simulink model "TV_2020_v1_TCELDAS_YAW_1_FUNregenerativa_ETAS"  (R2017b)
settings: Solver=ode3  StartTime=0  StopTime=10  FixedStep=0.05  RelTol=1e-3  EnableMultiTasking=on
(part 1 of 5)
settings Model: Creator=Manuel Montesinos  LastModifiedBy=Eric
settings DataIOCC: LimitDataPoints=on  SaveFormat=Array
settings OptimizationCC: LifeSpan=inf
settings DebuggingCC: SFUnexpectedBacktrackingDiag=warning  SFNoUnconditionalDefaultTransitionDiag=warning  SFExecutionAtInitializationDiag=none
settings HardwareCC: ProdBitPerPointer=32  ProdBitPerSizeT=32  ProdBitPerPtrDiffT=32  ProdLargestAtomicFloat=None  ProdIntDivRoundTo=Undefined  ProdEndianess=Unspecified  ProdWordSize=32  ProdHWDeviceType=32-bit Generic
settings ModelReferenceCC: PropagateSignalLabelsOutOfModel=off
settings CodeAppCC: StateflowObjectComments=on
settings GRTTargetCC: TargetLangStandard=C89/C90 (ANSI)
settings ConfigComp: CovMetricSettings=dw  CovSaveCumulativeToWorkspaceVar=on  CovSaveSingleToWorkspaceVar=on  CovExternalEMLEnable=off

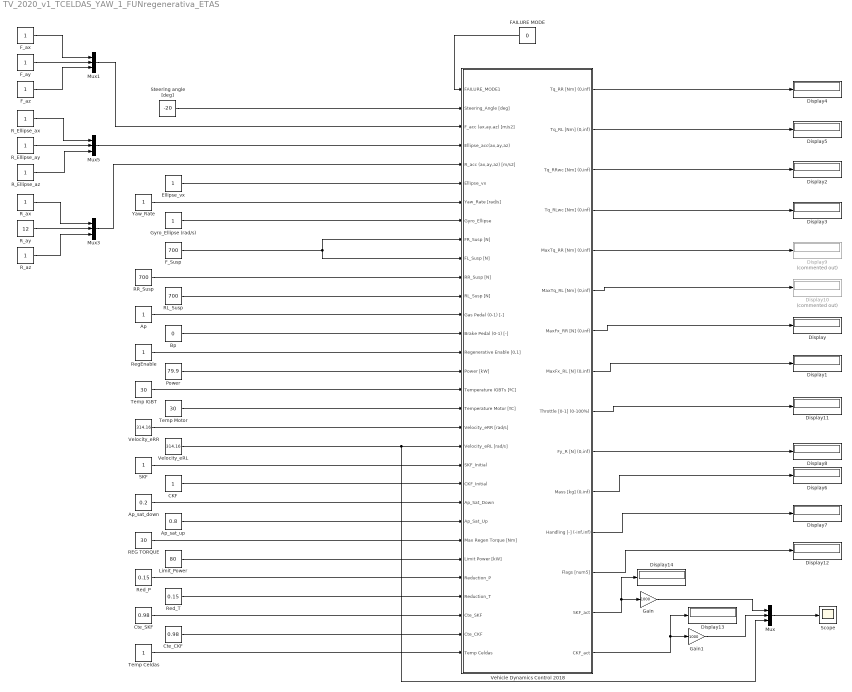
== system TV_2020_v1_TCELDAS_YAW_1_FUNregenerativa_ETAS ==
  Ap : Constant
  Ap_sat_down : Constant  Value=0.2
  Ap_sat_up : Constant  Value=0.8
  Bp : Constant  Value=0
  CKF : Constant
  Cte_CKF : Constant  Value=0.98
  Cte_SKF : Constant  Value=0.98
  Display{,1..8,11..14} (13 alike) : Display
  Display10 : Display  Commented=on
  Display9 : Display  Commented=on
  Ellipse_vx : Constant
  FAILURE MODE : Constant  Value=0
  F_Susp : Constant  Value=700
  F_ax : Constant
  F_ay : Constant
  F_az : Constant
  Gain : Gain  Gain=1000
  Gain1 : Gain  Gain=1000
  Gyro_Ellipse (rad/s) : Constant
  Limit_Power : Constant  Value=80
  Mux{,1,3,5} (4 alike) : Mux  Inputs=3
  Power : Constant  Value=79.9
  REG TORQUE : Constant  Value=30
  RL_Susp : Constant  Value=700
  RR_Susp : Constant  Value=700
  R_Ellipse_ax : Constant
  R_Ellipse_ay : Constant
  R_Ellipse_az : Constant
  R_ax : Constant
  R_ay : Constant  Value=12
  R_az : Constant
  Red_P : Constant  Value=0.15
  Red_T : Constant  Value=0.15
  RegEnable : Constant
  SKF : Constant
  Scope : Scope
  Steering angle [deg] : Constant  Value=-20
  Temp Celdas : Constant
  Temp IGBT : Constant  Value=30
  Temp Motor : Constant  Value=30
  Vehicle Dynamics Control 2018 : Subsystem
  Velocity_eRL : Constant  Value=314.16
  Velocity_eRR : Constant  Value=314.16
  Yaw_Rate : Constant
  wires:
  FAILURE MODE/1 -> Vehicle Dynamics Control 2018/1(FAILURE_MODE1)
  Vehicle Dynamics Control 2018/1(Tq_RR [Nm] (0,inf)) -> Display4/1
  Vehicle Dynamics Control 2018/2(Tq_RL [Nm] (0,inf)) -> Display5/1
  Mux3/1 -> Vehicle Dynamics Control 2018/5(R_acc (ax,ay,az) [m/s2])
  RegEnable/1 -> Vehicle Dynamics Control 2018/15(Regenerative Enable [0,1])
  Velocity_eRL/1 -> Vehicle Dynamics Control 2018/20(Velocity_eRL [rad/s]), Mux/3
  SKF/1 -> Vehicle Dynamics Control 2018/21(SKF_Initial)
  CKF/1 -> Vehicle Dynamics Control 2018/22(CKF_Initial)
  REG TORQUE/1 -> Vehicle Dynamics Control 2018/25(Max Regen Torque [Nm])
  Limit_Power/1 -> Vehicle Dynamics Control 2018/26(Limit Power [kW])
  Red_T/1 -> Vehicle Dynamics Control 2018/28(Reduction_T)
  Red_P/1 -> Vehicle Dynamics Control 2018/27(Reduction_P)
  F_Susp/1 -> Vehicle Dynamics Control 2018/9(FR_Susp [N]), Vehicle Dynamics Control 2018/10(FL_Susp [N])
  Vehicle Dynamics Control 2018/7(MaxFx_RR [N] (0,inf)) -> Display/1
  Vehicle Dynamics Control 2018/8(MaxFx_RL [N] (0,inf)) -> Display1/1
  Vehicle Dynamics Control 2018/3(Tq_RRwc [Nm] (0,inf)) -> Display2/1
  Vehicle Dynamics Control 2018/4(Tq_RLwc [Nm] (0,inf)) -> Display3/1
  Vehicle Dynamics Control 2018/6(MaxTq_RL [Nm] (0,inf)) -> Display10/1
  Vehicle Dynamics Control 2018/5(MaxTq_RR [Nm] (0,inf)) -> Display9/1
  Vehicle Dynamics Control 2018/10(Fy_R [N] (0,inf)) -> Display8/1
  Steering angle [deg]/1 -> Vehicle Dynamics Control 2018/2(Steering_Angle [deg])
  RR_Susp/1 -> Vehicle Dynamics Control 2018/11(RR_Susp [N])
  RL_Susp/1 -> Vehicle Dynamics Control 2018/12(RL_Susp [N])
  Bp/1 -> Vehicle Dynamics Control 2018/14(Brake Pedal (0-1) [-])
  Ap/1 -> Vehicle Dynamics Control 2018/13(Gas Pedal (0-1) [-])
  Ap_sat_down/1 -> Vehicle Dynamics Control 2018/23(Ap_Sat_Down)
  Vehicle Dynamics Control 2018/11(Mass [kg] (0,inf)) -> Display6/1
  Vehicle Dynamics Control 2018/12(Handling [-] (-inf,inf)) -> Display7/1
  Mux1/1 -> Vehicle Dynamics Control 2018/3(F_acc (ax,ay,az) [m/s2])
  Temp IGBT/1 -> Vehicle Dynamics Control 2018/17(Temperature IGBTs [ºC])
  Power/1 -> Vehicle Dynamics Control 2018/16(Power [kW])
  Temp Motor/1 -> Vehicle Dynamics Control 2018/18(Temperature Motor [ºC])
  Ap_sat_up/1 -> Vehicle Dynamics Control 2018/24(Ap_Sat_Up)
  Vehicle Dynamics Control 2018/9(Throttle [0-1] (0-100%)) -> Display11/1
  Vehicle Dynamics Control 2018/13(Flags [num5]) -> Display12/1
  Cte_SKF/1 -> Vehicle Dynamics Control 2018/29(Cte_SKF)
  Cte_CKF/1 -> Vehicle Dynamics Control 2018/30(Cte_CKF)
  Vehicle Dynamics Control 2018/15(CKF_act) -> Display13/1, Gain1/1
  Vehicle Dynamics Control 2018/14(SKF_act) -> Display14/1, Gain/1
  Mux/1 -> Scope/1
  Gain/1 -> Mux/1
  Gain1/1 -> Mux/2
  Yaw_Rate/1 -> Vehicle Dynamics Control 2018/7(Yaw_Rate [rad/s])
  F_ax/1 -> Mux1/1
  F_ay/1 -> Mux1/2
  F_az/1 -> Mux1/3
  R_ax/1 -> Mux3/1
  R_ay/1 -> Mux3/2
  R_az/1 -> Mux3/3
  Velocity_eRR/1 -> Vehicle Dynamics Control 2018/19(Velocity_eRR [rad/s])
  Mux5/1 -> Vehicle Dynamics Control 2018/4(Ellipse_acc(ax,ay,az))
  R_Ellipse_ay/1 -> Mux5/2
  R_Ellipse_ax/1 -> Mux5/1
  R_Ellipse_az/1 -> Mux5/3
  Ellipse_vx/1 -> Vehicle Dynamics Control 2018/6(Ellipse_vx)
  Gyro_Ellipse (rad/s)/1 -> Vehicle Dynamics Control 2018/8(Gyro_Ellipse)
  Temp Celdas/1 -> Vehicle Dynamics Control 2018/31(Temp Celdas)

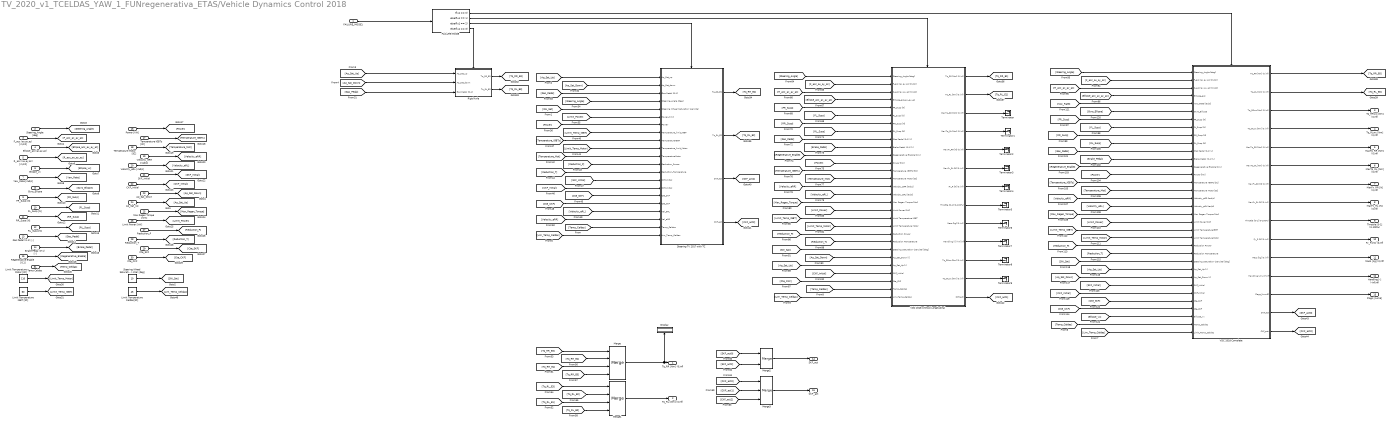
== system TV_2020_v1_TCELDAS_YAW_1_FUNregenerativa_ETAS/Vehicle Dynamics Control 2018 ==
  FAILURE_MODE1 : Inport
  Steering_Angle [deg] : Inport  Port=2
  F_acc (ax,ay,az) [m/s2] : Inport  Port=3
  Ellipse_acc(ax,ay,az) : Inport  Port=4
  R_acc (ax,ay,az) [m/s2] : Inport  Port=5
  Ellipse_vx : Inport  Port=6
  Yaw_Rate [rad/s] : Inport  Port=7
  Gyro_Ellipse : Inport  Port=8
  FR_Susp [N] : Inport  Port=9
  FL_Susp [N] : Inport  Port=10
  RR_Susp [N] : Inport  Port=11
  RL_Susp [N] : Inport  Port=12
  Gas Pedal (0-1) [-] : Inport  Port=13
  Brake Pedal (0-1) [-] : Inport  Port=14
  Regenerative Enable [0,1] : Inport  Port=15
  Power [kW] : Inport  Port=16
  Temperature IGBTs [ºC] : Inport  Port=17
  Temperature Motor [ºC] : Inport  Port=18
  Velocity_eRR [rad/s] : Inport  Port=19
  Velocity_eRL [rad/s] : Inport  Port=20
  SKF_Initial : Inport  Port=21
  CKF_Initial : Inport  Port=22
  Ap_Sat_Down : Inport  Port=23
  Ap_Sat_Up : Inport  Port=24
  Max Regen Torque [Nm] : Inport  Port=25
  Limit Power [kW] : Inport  Port=26
  Reduction_P : Inport  Port=27
  Reduction_T : Inport  Port=28
  Cte_SKF : Inport  Port=29
  Cte_CKF : Inport  Port=30
  Temp Celdas : Inport  Port=31
  Display : Display
  FAILURE MODE : If  IfExpression=u1 == 0  ElseIfExpressions=u1 == 1, u1 == 2, u1 == 3  ShowElse=off
  Limit Temperature Celdas[ºC] : Constant  Value=45
  Limit Temperature IGBT [ºC] : Constant  Value=60
  Limit Temperature Motor [ºC] : Constant  Value=110
  Merge : Merge  Inputs=4
  Merge1 : Merge  Inputs=4
  Merge2 : Merge
  Merge3 : Merge  Inputs=3
  Rigid Axle : Subsystem  TreatAsAtomicUnit=on
  Steering TV 2017 with TC : Subsystem  TreatAsAtomicUnit=on
  "Steering Wheel Saturation (per site) [deg] " : Constant  Value=10
  Terminator{,1..9} (10 alike) : Terminator
  VDC 2018 Complete : Subsystem  TreatAsAtomicUnit=on
  VDC 2018 without Longitudinal : Subsystem  TreatAsAtomicUnit=on
  Tq_RR [Nm] (0,inf) : Outport
  Tq_RL [Nm] (0,inf) : Outport  Port=2
  Tq_RRwc [Nm] (0,inf) : Outport  Port=3
  Tq_RLwc [Nm] (0,inf) : Outport  Port=4
  MaxTq_RR [Nm] (0,inf) : Outport  Port=5
  MaxTq_RL [Nm] (0,inf) : Outport  Port=6
  MaxFx_RR [N] (0,inf) : Outport  Port=7
  MaxFx_RL [N] (0,inf) : Outport  Port=8
  Throttle [0-1] (0-100%) : Outport  Port=9
  Fy_R [N] (0,inf) : Outport  Port=10
  Mass [kg] (0,inf) : Outport  Port=11
  Handling [-] (-inf,inf) : Outport  Port=12
  Flags [num5] : Outport  Port=13
  SKF_act : Outport  Port=14
  CKF_act : Outport  Port=15
  wires:
  Merge1/1 -> Tq_RL [Nm] (0,inf)/1
  Merge/1 -> Display/1, Tq_RR [Nm] (0,inf)/1
  Ap_Sat_Down/1 -> [Ap_Sat_Down]
  "Steering Wheel Saturation (per site) [deg] "/1 -> [SW_Sat]
  [Ap_Sat_Up] -> Rigid Axle/1("Ap_Sat_up ")
  [Ap_Sat_Down] -> Rigid Axle/2(Ap_Sat_down)
  VDC 2018 Complete/4(Tq_RLwc [Nm] (0,inf)) -> Tq_RLwc [Nm] (0,inf)/1
  VDC 2018 Complete/3(Tq_RRwc [Nm] (0,inf)) -> Tq_RRwc [Nm] (0,inf)/1
  VDC 2018 Complete/5(MaxTq_RR [Nm] (0,inf)) -> MaxTq_RR [Nm] (0,inf)/1
  VDC 2018 Complete/6(MaxTq_RL [Nm] (0,inf)) -> MaxTq_RL [Nm] (0,inf)/1
  VDC 2018 Complete/7(MaxFx_RR [N] (0,inf)) -> MaxFx_RR [N] (0,inf)/1
  VDC 2018 Complete/8(MaxFx_RL [N] (0,inf)) -> MaxFx_RL [N] (0,inf)/1
  VDC 2018 Complete/9(Throttle [0-1] (0-100%)) -> Throttle [0-1] (0-100%)/1
  VDC 2018 Complete/10(Fy_R [N] (0,inf)) -> Fy_R [N] (0,inf)/1
  VDC 2018 Complete/11(Mass [kg] (0,inf)) -> Mass [kg] (0,inf)/1
  VDC 2018 Complete/12(Handling [-] (-inf,inf)) -> Handling [-] (-inf,inf)/1
  VDC 2018 without Longitudinal/3(MaxTq_RR [Nm] (0,inf)) -> Terminator/1
  VDC 2018 without Longitudinal/4(MaxTq_RL [Nm] (0,inf)) -> Terminator1/1
  VDC 2018 without Longitudinal/5(MaxFx_RR [N] (0,inf)) -> Terminator2/1
  VDC 2018 without Longitudinal/6(MaxFx_RL [N] (0,inf)) -> Terminator3/1
  VDC 2018 without Longitudinal/7(Fy_R [N] (0,inf)) -> Terminator4/1
  VDC 2018 without Longitudinal/8(Throttle [0-1] (0-100%)) -> Terminator5/1
  VDC 2018 without Longitudinal/9(Mass [kg] (0,inf)) -> Terminator6/1
  VDC 2018 without Longitudinal/10(Handling [-] (-inf,inf)) -> Terminator7/1
  VDC 2018 without Longitudinal/11(Tq_RRwc [Nm] (0,inf)) -> Terminator8/1
  VDC 2018 without Longitudinal/12(Tq_RLwc [Nm] (0,inf)) -> Terminator9/1
  Ap_Sat_Up/1 -> [Ap_Sat_Up]
  VDC 2018 Complete/13(Flags_[num5]) -> Flags [num5]/1
  Merge2/1 -> SKF_act/1
  Merge3/1 -> CKF_act/1
  Steering_Angle [deg]/1 -> [Steering_Angle]
  F_acc (ax,ay,az) [m/s2]/1 -> [F_acc_ax_ay_az]
  Ellipse_acc(ax,ay,az)/1 -> [Ellipse_acc_ax_ay_az]
  R_acc (ax,ay,az) [m/s2]/1 -> [R_acc_ax_ay_az]
  Ellipse_vx/1 -> [Ellipse_vx]
  Yaw_Rate [rad/s]/1 -> [Yaw_Rate]
  Gyro_Ellipse/1 -> [Gyro_Ellipse]
  FR_Susp [N]/1 -> [FR_Susp]
  FL_Susp [N]/1 -> [FL_Susp]
  RR_Susp [N]/1 -> [RR_Susp]
  RL_Susp [N]/1 -> [RL_Susp]
  Gas Pedal (0-1) [-]/1 -> [Gas_Pedal]
  Brake Pedal (0-1) [-]/1 -> [Brake_Pedal]
  Regenerative Enable [0,1]/1 -> [Regenerative_Enable]
  Power [kW]/1 -> [Power]
  Temperature IGBTs [ºC]/1 -> [Temperature_IGBTs]
  Temperature Motor [ºC]/1 -> [Temperature_Mot]
  Velocity_eRR [rad/s]/1 -> [Velocity_eRR]
  Velocity_eRL [rad/s]/1 -> [Velocity_eRL]
  SKF_Initial/1 -> [SKF_Initial]
  CKF_Initial/1 -> [CKF_Initial]
  Max Regen Torque [Nm]/1 -> [Max_Regen_Torque]
  Limit Power [kW]/1 -> [Limit_Power]
  Reduction_P/1 -> [Reduction_P]
  Reduction_T/1 -> [Reduction_T]
  Cte_SKF/1 -> [Cte_SKF]
  Cte_CKF/1 -> [Cte_CKF]
  [Gas_Pedal] -> Rigid Axle/3(Gas Pedal [0-1])
  [Ap_Sat_Up] -> Steering TV 2017 with TC/1("Ap_Sat_up ")
  [Ap_Sat_Down] -> Steering TV 2017 with TC/2(Ap_Sat_down)
  [Gas_Pedal] -> Steering TV 2017 with TC/3(Gas Pedal [0-1])
  [Steering_Angle] -> Steering TV 2017 with TC/4(Steering_Angle [deg])
  [SW_Sat] -> Steering TV 2017 with TC/5("Steering Wheel Saturation (per site) ")
  [Limit_Power] -> Steering TV 2017 with TC/6(Power_limit)
  [Power] -> Steering TV 2017 with TC/7(Power)
  Limit Temperature Motor [ºC]/1 -> [Limit_Temp_Motor]
  Limit Temperature IGBT [ºC]/1 -> [Limit_Temp_IGBT]
  [Limit_Temp_Motor] -> Steering TV 2017 with TC/10(Temperature_limit_Motor)
  [Limit_Temp_IGBT] -> Steering TV 2017 with TC/8(Temperature_limit_IGBT)
  [Temperature_IGBTs] -> Steering TV 2017 with TC/9(TemperatureIGBT)
  [Temperature_Mot] -> Steering TV 2017 with TC/11(TemperatureMotor)
  [Reduction_P] -> Steering TV 2017 with TC/12(Reduction_Power)
  [Reduction_T] -> Steering TV 2017 with TC/13(Reduction_Temperature)
  [SKF_Initial] -> Steering TV 2017 with TC/14(SKF_Initial)
  [CKF_Initial] -> Steering TV 2017 with TC/15(CKF_Initial)
  [Cte_SKF] -> Steering TV 2017 with TC/16(Cte_SKF)
  [Cte_CKF] -> Steering TV 2017 with TC/17(Cte_CKF)
  [Velocity_eRL] -> Steering TV 2017 with TC/18(Vel_eRL)
  [Velocity_eRR] -> Steering TV 2017 with TC/19(Vel_eRR)
  Rigid Axle/1(Tq_RR_E3) -> [Tq_RR_E3]
  Rigid Axle/2(Tq_RL_E3) -> [Tq_RL_E3]
  [Tq_RL_E3] -> Merge1/1
  [Tq_RR_E3] -> Merge/1
  Steering TV 2017 with TC/1(Tq_RR_E2) -> [Tq_RR_E2]
  Steering TV 2017 with TC/2(Tq_RL_E2) -> [Tq_RL_E2]
  [Tq_RL_E2] -> Merge1/2
  [Tq_RR_E2] -> Merge/2
  VDC 2018 without Longitudinal/2(Tq_RL [Nm] (0,inf)) -> [Tq_RL_E1]
  VDC 2018 without Longitudinal/1(Tq_RR [Nm] (0,inf)) -> [Tq_RR_E1]
  [Tq_RR_E1] -> Merge/3
  [Tq_RL_E1] -> Merge1/3
  VDC 2018 Complete/1(Tq_RR [Nm] (0,inf)) -> [Tq_RR_E0]
  VDC 2018 Complete/2(Tq_RL [Nm] (0,inf)) -> [Tq_RL_E0]
  [Tq_RR_E0] -> Merge/4
  [Tq_RL_E0] -> Merge1/4
  Steering TV 2017 with TC/3(SKF_act) -> [SKF_act2]
  Steering TV 2017 with TC/4(CKF_act) -> [CKF_act2]
  VDC 2018 without Longitudinal/13(CKF_act) -> [CKF_act1]
  VDC 2018 Complete/14(SKF_act) -> [SKF_act0]
  VDC 2018 Complete/15(CKF_act) -> [CKF_act0]
  [CKF_act1] -> Merge3/2
  [CKF_act0] -> Merge3/1
  [CKF_act2] -> Merge3/3
  [SKF_act0] -> Merge2/1
  [SKF_act2] -> Merge2/2
  [Steering_Angle] -> VDC 2018 without Longitudinal/1(Steering_Angle [deg])
  [F_acc_ax_ay_az] -> VDC 2018 without Longitudinal/2(F_acc (ax,ay,az) [m/s2])
  [Ellipse_acc_ax_ay_az] -> VDC 2018 without Longitudinal/4(Ellipse_acc_ax_ay_az)
  [R_acc_ax_ay_az] -> VDC 2018 without Longitudinal/3(R_acc (ax,ay,az) [m/s2])
  [FR_Susp] -> VDC 2018 without Longitudinal/5(FR_Susp [N])
  [FL_Susp] -> VDC 2018 without Longitudinal/6(FL_Susp [N])
  [RR_Susp] -> VDC 2018 without Longitudinal/7(RR_Susp [N])
  [RL_Susp] -> VDC 2018 without Longitudinal/8(RL_Susp [N])
  [Gas_Pedal] -> VDC 2018 without Longitudinal/9(Gas Pedal (0-1) [-])
  [Brake_Pedal] -> VDC 2018 without Longitudinal/10(Brake Pedal (0-1) [-])
  [Regenerative_Enable] -> VDC 2018 without Longitudinal/11(Regenerative Enable [0,1])
  [Power] -> VDC 2018 without Longitudinal/12(Power [kW])
  [Temperature_IGBTs] -> VDC 2018 without Longitudinal/13(Temperature IGBTs [ºC])
  [Temperature_Mot] -> VDC 2018 without Longitudinal/14(Temperature Motor [ºC])
  [Velocity_eRR] -> VDC 2018 without Longitudinal/15(Velocity_eRR [rad/s])
  [Velocity_eRL] -> VDC 2018 without Longitudinal/16(Velocity_eRL [rad/s])
  [Max_Regen_Torque] -> VDC 2018 without Longitudinal/17(Max Regen Torque [Nm])
  [Limit_Power] -> VDC 2018 without Longitudinal/18(Limit Power [kW])
  [Limit_Temp_IGBT] -> VDC 2018 without Longitudinal/19(Limit Temperature IGBT)
  [Limit_Temp_Motor] -> VDC 2018 without Longitudinal/20(Limit Temperature Motor)
  [Cte_CKF] -> VDC 2018 without Longitudinal/27(Cte_CKF)
  [Reduction_P] -> VDC 2018 without Longitudinal/21(Reduction Power)
  [Reduction_T] -> VDC 2018 without Longitudinal/22(Reduction Temperature)
  [Ap_Sat_Up] -> VDC 2018 without Longitudinal/25(Ap_Sat_Up [-])
  [Ap_Sat_Down] -> VDC 2018 without Longitudinal/24(Ap_Sat_Down [-])
  [SW_Sat] -> VDC 2018 without Longitudinal/23(Steering Saturation (per site) [deg])
  [CKF_Initial] -> VDC 2018 without Longitudinal/26(CKF_Initial)
  [Steering_Angle] -> VDC 2018 Complete/1(Steering_Angle [deg])
  [F_acc_ax_ay_az] -> VDC 2018 Complete/2(F_acc (ax,ay,az) [m/s2])
  [R_acc_ax_ay_az] -> VDC 2018 Complete/3(R_acc (ax,ay,az) [m/s2])
  [Ellipse_acc_ax_ay_az] -> VDC 2018 Complete/4(Ellipse_acc)
  [FR_Susp] -> VDC 2018 Complete/7(FR_Susp [N])
  [FL_Susp] -> VDC 2018 Complete/8(FL_Susp [N])
  [RR_Susp] -> VDC 2018 Complete/9(RR_Susp [N])
  [RL_Susp] -> VDC 2018 Complete/10(RL_Susp [N])
  [Gas_Pedal] -> VDC 2018 Complete/11(Gas Pedal (0-1) [-])
  [Brake_Pedal] -> VDC 2018 Complete/12(Brake Pedal (0-1) [-])
  [Power] -> VDC 2018 Complete/14(Power [kW])
  [Regenerative_Enable] -> VDC 2018 Complete/13(Regenerative Enable [0,1])
  [Temperature_IGBTs] -> VDC 2018 Complete/15(Temperature IGBTs [ºC])
  [Temperature_Mot] -> VDC 2018 Complete/16(Temperature Motor [ºC])
  [Velocity_eRR] -> VDC 2018 Complete/17(Velocity_eRR [rad/s])
  [Velocity_eRL] -> VDC 2018 Complete/18(Velocity_eRL [rad/s])
  [Max_Regen_Torque] -> VDC 2018 Complete/19(Max Regen Torque [Nm])
  [Limit_Power] -> VDC 2018 Complete/20(Limit Power [kW])
  [Limit_Temp_IGBT] -> VDC 2018 Complete/21(Limit TemperatureIGBT)
  [Limit_Temp_Motor] -> VDC 2018 Complete/22(Limit TemperatureMotor)
  [Reduction_P] -> VDC 2018 Complete/23(Reduction Power)
  [Reduction_T] -> VDC 2018 Complete/24(Reduction Temperature)
  [SW_Sat] -> VDC 2018 Complete/25(Steering Saturation (per site) [deg])
  [Ap_Sat_Down] -> VDC 2018 Complete/27(Ap_Sat_Down [-])
  [Ap_Sat_Up] -> VDC 2018 Complete/26(Ap_Sat_Up [-])
  [CKF_Initial] -> VDC 2018 Complete/29(CKF_Initial)
  [Yaw_Rate] -> VDC 2018 Complete/5(Yaw_Rate [rad/s])
  [Gyro_Ellipse] -> VDC 2018 Complete/6(Gyro_Ellipse)
  [Cte_CKF] -> VDC 2018 Complete/31(Cte_CKF)
  [Cte_SKF] -> VDC 2018 Complete/30(Cte_SKF)
  [SKF_Initial] -> VDC 2018 Complete/28(SKF_Initial)
  [Ellipse_vx] -> VDC 2018 Complete/32(Ellipse_vx)
  FAILURE MODE/1 -> VDC 2018 Complete/Action
  FAILURE_MODE1/1 -> FAILURE MODE/1
  FAILURE MODE/2 -> VDC 2018 without Longitudinal/Action
  FAILURE MODE/3 -> Steering TV 2017 with TC/Action
  FAILURE MODE/4 -> Rigid Axle/Action
  Temp Celdas/1 -> [Temp_Celdas]
  Limit Temperature Celdas[ºC]/1 -> [Lim_Temp_Celdas]
  [Temp_Celdas] -> Steering TV 2017 with TC/20(Temp_Celdas)
  [Lim_Temp_Celdas] -> Steering TV 2017 with TC/21(Lim_Temp_Celdas)
  [Temp_Celdas] -> VDC 2018 without Longitudinal/28(Temp_Celdas)
  [Lim_Temp_Celdas] -> VDC 2018 without Longitudinal/29(Lim_Temp_Celdas)
  [Temp_Celdas] -> VDC 2018 Complete/33(Temp_Celdas)
  [Lim_Temp_Celdas] -> VDC 2018 Complete/34(Limit_Temp_Celdas)

== system TV_2020_v1_TCELDAS_YAW_1_FUNregenerativa_ETAS/Vehicle Dynamics Control 2018/Rigid Axle ==
  "Ap_Sat_up " : Inport
  Ap_Sat_down : Inport  Port=2
  Gas Pedal [0-1] : Inport  Port=3
  Action Port : ActionPort
  Accelerating : Subsystem
  Torque_RL [Nm] : Constant  Value=60
  Torque_RR [Nm] : Constant  Value=60
  Tq_RR_E3 : Outport
  Tq_RL_E3 : Outport  Port=2
  wires:
  Torque_RR [Nm]/1 -> Accelerating/4(Tq_RR)
  Torque_RL [Nm]/1 -> Accelerating/5("Tq_RL ")
  Accelerating/2(Tq_RL) -> Tq_RL_E3/1
  Accelerating/1("Tq_RR ") -> Tq_RR_E3/1
  Gas Pedal [0-1]/1 -> Accelerating/1(Ap)
  "Ap_Sat_up "/1 -> Accelerating/2("Ap_Sat_up ")
  Ap_Sat_down/1 -> Accelerating/3(Ap_Sat_down)

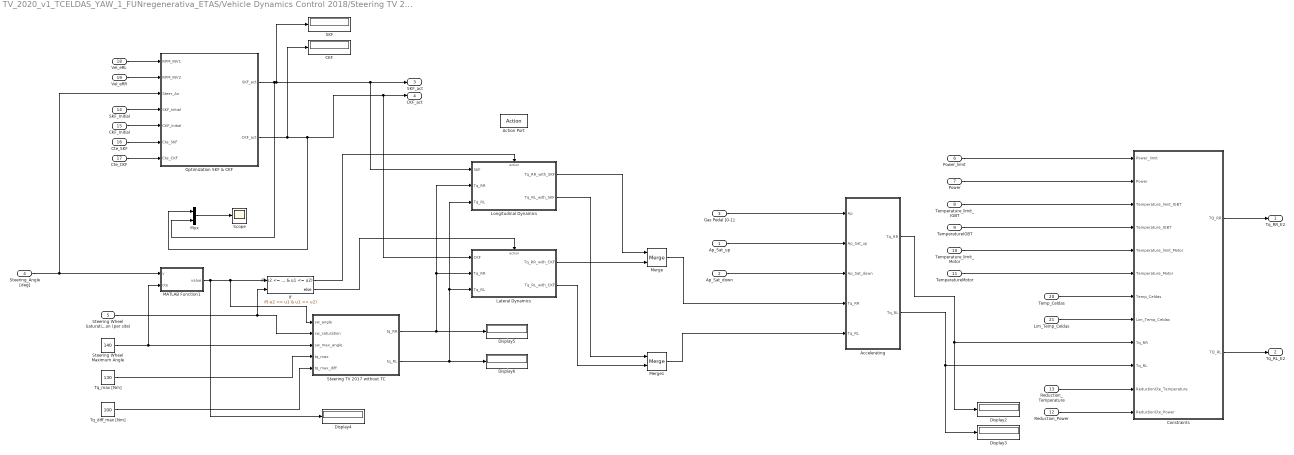
== system TV_2020_v1_TCELDAS_YAW_1_FUNregenerativa_ETAS/Vehicle Dynamics Control 2018/Steering TV 2017 with TC ==
  "Ap_Sat_up " : Inport
  Ap_Sat_down : Inport  Port=2
  Gas Pedal [0-1] : Inport  Port=3
  Steering_Angle [deg] : Inport  Port=4
  "Steering Wheel Saturation (per site) " : Inport  Port=5
  Power_limit : Inport  Port=6
  Power : Inport  Port=7
  Temperature_limit_IGBT : Inport  Port=8
  TemperatureIGBT : Inport  Port=9
  Temperature_limit_Motor : Inport  Port=10
  TemperatureMotor : Inport  Port=11
  Reduction_Power : Inport  Port=12
  Reduction_Temperature : Inport  Port=13
  SKF_Initial : Inport  Port=14
  CKF_Initial : Inport  Port=15
  Cte_SKF : Inport  Port=16
  Cte_CKF : Inport  Port=17
  Vel_eRL : Inport  Port=18
  Vel_eRR : Inport  Port=19
  Temp_Celdas : Inport  Port=20
  Lim_Temp_Celdas : Inport  Port=21
  Action Port : ActionPort
  Accelerating : Subsystem
  CKF : Display
  Constraints : Subsystem
  Display{2..6} (5 alike) : Display
  If : If  NumInputs=2  IfExpression=-u2 <= u1 & u1 <= u2
  Lateral Dynamics : Subsystem  TreatAsAtomicUnit=on
  Longitudinal Dynamics : Subsystem  TreatAsAtomicUnit=on
  MATLAB Function1 : MATLAB Function  TreatAsAtomicUnit=on
  Merge : Merge
  Merge1 : Merge
  Mux : Mux  Inputs=2
  Optimization SKF & CKF : Subsystem
  SKF : Display
  Scope : Scope
  Steering TV 2017 without TC : MATLAB Function  TreatAsAtomicUnit=on
  Steering Wheel Maximum Angle : Constant  Value=140
  Tq_diff_max [Nm] : Constant  Value=100
  Tq_max [Nm] : Constant  Value=130
  Tq_RR_E2 : Outport
  Tq_RL_E2 : Outport  Port=2
  SKF_act : Outport  Port=3
  CKF_act : Outport  Port=4
  wires:
  Gas Pedal [0-1]/1 -> Accelerating/1(Ap)
  "Ap_Sat_up "/1 -> Accelerating/2("Ap_Sat_up ")
  Ap_Sat_down/1 -> Accelerating/3(Ap_Sat_down)
  Tq_max [Nm]/1 -> Steering TV 2017 without TC/4(tq_max)
  Tq_diff_max [Nm]/1 -> Steering TV 2017 without TC/5(tq_max_diff)
  Steering Wheel Maximum Angle/1 -> Steering TV 2017 without TC/3(sw_max_angle), MATLAB Function1/2(cte)
  "Steering Wheel Saturation (per site) "/1 -> If/2, Steering TV 2017 without TC/2(sw_saturation)
  Steering TV 2017 without TC/1(tq_RR) -> Display5/1, Longitudinal Dynamics/2(Tq_RR), Lateral Dynamics/2(Tq_RR)
  Steering TV 2017 without TC/2(tq_RL) -> Longitudinal Dynamics/3(Tq_RL), Lateral Dynamics/3(Tq_RL), Display6/1
  Power_limit/1 -> Constraints/1(Power_limit)
  Power/1 -> Constraints/2(Power)
  Temperature_limit_IGBT/1 -> Constraints/3(Temperature_limit_IGBT)
  TemperatureIGBT/1 -> Constraints/4(Temperature_IGBT)
  Reduction_Temperature/1 -> Constraints/11(ReductionCte_Temperature)
  Reduction_Power/1 -> Constraints/12(ReductionCte_Power)
  Constraints/1(TQ_RR) -> Tq_RR_E2/1
  Constraints/2(TQ_RL) -> Tq_RL_E2/1
  Accelerating/2(Tq_RL) -> Display3/1, Constraints/10(Tq_RL)
  Accelerating/1("Tq_RR ") -> Display2/1, Constraints/9(Tq_RR)
  MATLAB Function1/1(value) -> Display4/1, Steering TV 2017 without TC/1(sw_angle), If/1
  Temperature_limit_Motor/1 -> Constraints/5(Temperature_limit_Motor)
  TemperatureMotor/1 -> Constraints/6(Temperature_Motor)
  Optimization SKF & CKF/2(CKF_act) -> CKF/1, Mux/1, Lateral Dynamics/1(CKF), CKF_act/1
  SKF_Initial/1 -> Optimization SKF & CKF/4(SKF_Initial)
  Mux/1 -> Scope/1
  Cte_SKF/1 -> Optimization SKF & CKF/6(Cte_SKF)
  Vel_eRL/1 -> Optimization SKF & CKF/1(RPM_INV1)
  Vel_eRR/1 -> Optimization SKF & CKF/2(RPM_INV2)
  Optimization SKF & CKF/1(SKF_act) -> SKF_act/1, Longitudinal Dynamics/1(SKF), SKF/1, Mux/2
  Steering_Angle [deg]/1 -> MATLAB Function1/1(v), Optimization SKF & CKF/3(Steer_An)
  CKF_Initial/1 -> Optimization SKF & CKF/5(CKF_Initial)
  Cte_CKF/1 -> Optimization SKF & CKF/7(Cte_CKF)
  If/1 -> Longitudinal Dynamics/Action
  Lateral Dynamics/2(Tq_RL_with_CKF) -> Merge1/2
  If/2 -> Lateral Dynamics/Action
  Longitudinal Dynamics/2(Tq_RL_with_SKF) -> Merge1/1
  Longitudinal Dynamics/1(Tq_RR_with_SKF) -> Merge/1
  Lateral Dynamics/1(Tq_RR_with_CKF) -> Merge/2
  Merge/1 -> Accelerating/4(Tq_RR)
  Merge1/1 -> Accelerating/5("Tq_RL ")
  Temp_Celdas/1 -> Constraints/7(Temp_Celdas)
  Lim_Temp_Celdas/1 -> Constraints/8(Lim_Temp_Celdas)

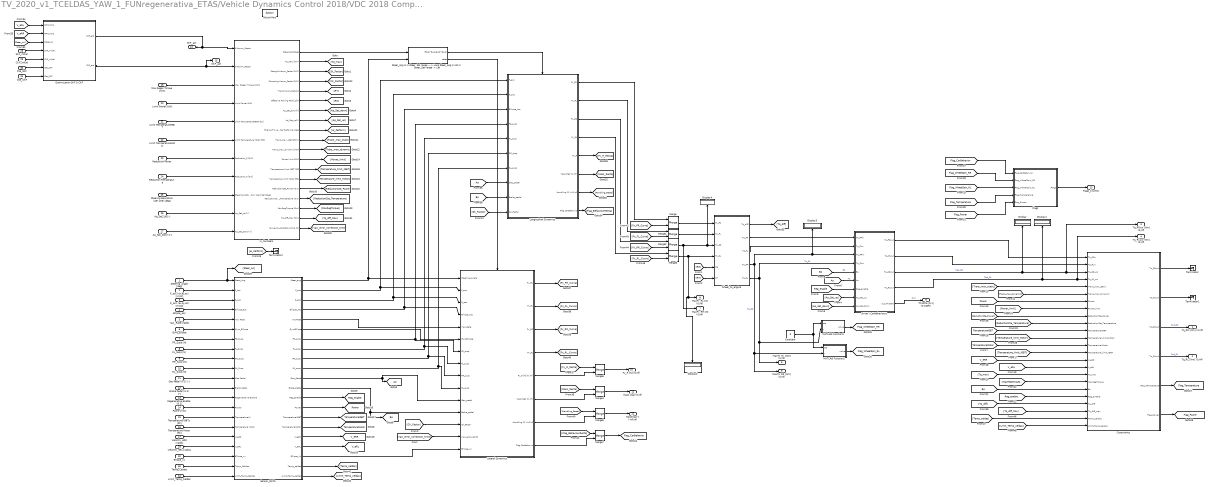
== system TV_2020_v1_TCELDAS_YAW_1_FUNregenerativa_ETAS/Vehicle Dynamics Control 2018/VDC 2018 Complete ==
  Steering_Angle [deg] : Inport
  F_acc (ax,ay,az) [m/s2] : Inport  Port=2
  R_acc (ax,ay,az) [m/s2] : Inport  Port=3
  Ellipse_acc : Inport  Port=4
  Yaw_Rate [rad/s] : Inport  Port=5
  Gyro_Ellipse : Inport  Port=6
  FR_Susp [N] : Inport  Port=7
  FL_Susp [N] : Inport  Port=8
  RR_Susp [N] : Inport  Port=9
  RL_Susp [N] : Inport  Port=10
  Gas Pedal (0-1) [-] : Inport  Port=11
  Brake Pedal (0-1) [-] : Inport  Port=12
  Regenerative Enable [0,1] : Inport  Port=13
  Power [kW] : Inport  Port=14
  Temperature IGBTs [ºC] : Inport  Port=15
  Temperature Motor [ºC] : Inport  Port=16
  Velocity_eRR [rad/s] : Inport  Port=17
  Velocity_eRL [rad/s] : Inport  Port=18
  Max Regen Torque [Nm] : Inport  Port=19
  Limit Power [kW] : Inport  Port=20
  Limit TemperatureIGBT : Inport  Port=21
  Limit TemperatureMotor : Inport  Port=22
  Reduction Power : Inport  Port=23
  Reduction Temperature : Inport  Port=24
  Steering Saturation (per site) [deg] : Inport  Port=25
  Ap_Sat_Up [-] : Inport  Port=26
  Ap_Sat_Down [-] : Inport  Port=27
  SKF_Initial : Inport  Port=28
  CKF_Initial : Inport  Port=29
  Cte_SKF : Inport  Port=30
  Cte_CKF : Inport  Port=31
  Ellipse_vx : Inport  Port=32
  Temp_Celdas : Inport  Port=33
  Limit_Temp_Celdas : Inport  Port=34
  Action Port : ActionPort
  Constant : Constant  Value=0
  Constraints : Subsystem
  Display{,1..4} (5 alike) : Display
  Driver / CarBehaviours : Subsystem
  Flags : Subsystem
  In_Numbers : Subsystem
  Lateral Dynamics : Subsystem  TreatAsAtomicUnit=on
  Longitudinal Dynamics : Subsystem  TreatAsAtomicUnit=on
  MATLAB Function1 : MATLAB Function  TreatAsAtomicUnit=on
  MATLAB Function2 : MATLAB Function  TreatAsAtomicUnit=on
  Merge{,1..7} (8 alike) : Merge
  Optimization SKF & CKF : Subsystem
  Sensor_DATA : Subsystem
  "Steer_ang is in Steer_Sat range ---> Long Steer_ang is not in Steer_Sat range -> Lat " : If  NumInputs=2  IfExpression=u2>=-u1&u2<=u1
  Terminator : Terminator
  Terminator1 : Terminator
  Terminator2 : Terminator
  Wheel_to_engine : Subsystem
  Tq_RR [Nm] (0,inf) : Outport
  Tq_RL [Nm] (0,inf) : Outport  Port=2
  Tq_RRwc [Nm] (0,inf) : Outport  Port=3
  Tq_RLwc [Nm] (0,inf) : Outport  Port=4
  MaxTq_RR [Nm] (0,inf) : Outport  Port=5
  MaxTq_RL [Nm] (0,inf) : Outport  Port=6
  MaxFx_RR [N] (0,inf) : Outport  Port=7
  MaxFx_RL [N] (0,inf) : Outport  Port=8
  Throttle [0-1] (0-100%) : Outport  Port=9
  Fy_R [N] (0,inf) : Outport  Port=10
  Mass [kg] (0,inf) : Outport  Port=11
  Handling [-] (-inf,inf) : Outport  Port=12
  Flags_[num5] : Outport  Port=13
  SKF_act : Outport  Port=14
  CKF_act : Outport  Port=15
  tag scope: Ap=global, Bp=global, Flag_CarBehavior=global, Flag_Power=global, Flag_Temperature=global, Flag_WheelSpin_RL=global, Flag_WheelSpin_RR=global, Power=global, Reg_enable=global, TemperatureIGBT=global, TemperatureMotor=global, V_eRL=global, V_eRR=global
  wires:
  "Steer_ang is in Steer_Sat range ---> Long Steer_ang is not in Steer_Sat range -> Lat "/1 -> Longitudinal Dynamics/Action
  "Steer_ang is in Steer_Sat range ---> Long Steer_ang is not in Steer_Sat range -> Lat "/2 -> Lateral Dynamics/Action
  Sensor_DATA/10(RL_susp) -> Lateral Dynamics/10(RL_susp), Longitudinal Dynamics/7(RL_susp)
  In_Numbers/3(Straight Kamm_Factor [0-2]) -> [SK_Factor]
  In_Numbers/1(Steer_Sat [deg]) -> "Steer_ang is in Steer_Sat range ---> Long Steer_ang is not in Steer_Sat range -> Lat "/1
  In_Numbers/2(Tq_Max [Nm]) -> [Tq_max]
  Sensor_DATA/11(Gas_Pedal) -> [Ap], Lateral Dynamics/11(Gas_pedal)
  In_Numbers/6(Effective Rolling Radius[m]) -> [Re]
  In_Numbers/5(Transmision_Ratio[-]) -> [RT]
  Sensor_DATA/9(RR_susp) -> Lateral Dynamics/9(RR_susp), Longitudinal Dynamics/6(RR_susp)
  In_Numbers/8(Ap_Sat_up[-]) -> [Ap_Sat_up]
  In_Numbers/7(Ap_Sat_down[-]) -> [Ap_Sat_down]
  Driver / CarBehaviours/3(Tq_RRout) -> Tq_RRwc [Nm] (0,inf)/1, Constraints/3(Tq_RR_wc), Display/1  "Teo_RR"
  Sensor_DATA/2(F_acc) -> Lateral Dynamics/2(F_acc), Longitudinal Dynamics/1(F_acc)
  Sensor_DATA/3(R_acc) -> Lateral Dynamics/3(R_acc), Longitudinal Dynamics/2(R_acc)
  Sensor_DATA/12(Brake_Pedal) -> [Bp], Lateral Dynamics/12(Brake_pedal)
  Sensor_DATA/8(FL_susp) -> Lateral Dynamics/8(FL_susp), Longitudinal Dynamics/5(FL_susp)
  Sensor_DATA/13(Reg_Enable) -> [Reg_enable]
  Sensor_DATA/7(FR_susp) -> Lateral Dynamics/7(FR_susp), Longitudinal Dynamics/4(FR_susp)
  Sensor_DATA/1(Steer_ang) -> "Steer_ang is in Steer_Sat range ---> Long Steer_ang is not in Steer_Sat range -> Lat "/2, Lateral Dynamics/1(Steering_Angle)
  Wheel_to_engine/5(Tq_RL) -> Driver / CarBehaviours/4("Tq_RLin "), MaxTq_RL [Nm] (0,inf)/1, MATLAB Function1/2(v)  "Tq_RL"
  [Trans_max_dynamic] -> Constraints/6(Trans_max_dynamic)
  [Power_limit] -> Constraints/8(Power_limit)
  In_Numbers/15(ReductionCte_Power (0-1)) -> [ReductionCte_Power]
  Driver / CarBehaviours/5(out_Throttle) -> Throttle [0-1] (0-100%)/1  "Out"
  Wheel_to_engine/4(Tq_RR) -> Driver / CarBehaviours/3(Tq_RRin), Display3/1, MaxTq_RR [Nm] (0,inf)/1, MATLAB Function2/2(v)  "Tq_RR"
  Wheel_to_engine/3(Tq_FL) -> Driver / CarBehaviours/2(Tq_FLin)
  In_Numbers/11(Trans_max_dynamic [Nm]) -> [Trans_max_dynamic]
  [Reg_enable] -> Driver / CarBehaviours/7(Reg_enable)
  [ReductionCte_Power] -> Constraints/9(ReductionCte_Power)
  [Ap_Sat_up] -> Driver / CarBehaviours/8(Ap_Sat_up)
  In_Numbers/10(Trans_max _static[Nm]) -> [Trans_max_static]
  [Ap] -> Driver / CarBehaviours/6(Ap)  "Ap"
  [Power] -> Constraints/7(Power)
  In_Numbers/12("Power limit [KW] ") -> [Power_limit]
  [Ap_Sat_down] -> Driver / CarBehaviours/9(Ap_Sat_down)
  Driver / CarBehaviours/4(Tq_RLout) -> Tq_RLwc [Nm] (0,inf)/1, Constraints/4("Tq_RL_wc "), Display1/1  "Teo_RL"
  Driver / CarBehaviours/2("Tq_FLout ") -> Constraints/2(Tq_FLin)
  Steering_Angle [deg]/1 -> [Steer_An], Sensor_DATA/1(Steer_Ang)
  Wheel_to_engine/2(Tq_FR) -> Driver / CarBehaviours/1(Tq_FRin)
  Driver / CarBehaviours/1(Tq_FRout) -> Constraints/1(Tq_FRin)
  [Trans_max_static] -> Constraints/5("Trans_max_static ")
  [Temperature_limit_IGBT] -> Constraints/14(Temperature_limit_IGBT)
  [Bp] -> Constraints/19(Bp)
  Sensor_DATA/18(V_eRL) -> [V_eRL]
  In_Numbers/17(MaxRegTorque [Nm]) -> [MaxRegTorque]
  [TemperatureIGBT] -> Constraints/11(TemperatureIGBT)
  [Reg_enable] -> Constraints/20(Reg_enable)
  In_Numbers/9(Engine+Inverter Performance[-]) -> [ei_Perform]
  [Bp] -> Driver / CarBehaviours/5(Bp)  "Bp"
  [Tq_max] -> Constraints/17(Tq_max)
  RR_Susp [N]/1 -> Sensor_DATA/9(RR_Susp)
  Power [kW]/1 -> Sensor_DATA/14("Power ")
  Sensor_DATA/14(Power) -> [Power]
  Sensor_DATA/17("V_eRR ") -> [V_eRR]
  [V_eRR] -> Constraints/15(V_eRR)
  Regenerative Enable [0,1]/1 -> Sensor_DATA/13(Regenerative Enable)
  Brake Pedal (0-1) [-]/1 -> Sensor_DATA/12(Brake Pedal)
  [V_eRL] -> Constraints/16(V_eRL)
  In_Numbers/13(Temperature limit IGBT [ºC]) -> [Temperature_limit_IGBT]
  FL_Susp [N]/1 -> Sensor_DATA/8(FL_Susp)
  FR_Susp [N]/1 -> Sensor_DATA/7(FR_Susp)
  R_acc (ax,ay,az) [m/s2]/1 -> Sensor_DATA/3(R_Acc)
  F_acc (ax,ay,az) [m/s2]/1 -> Sensor_DATA/2("F_Acc ")
  RL_Susp [N]/1 -> Sensor_DATA/10(RL_Susp)
  Gas Pedal (0-1) [-]/1 -> Sensor_DATA/11(Gas Pedal)
  Temperature IGBTs [ºC]/1 -> Sensor_DATA/15(TemperatureIN)
  Velocity_eRR [rad/s]/1 -> Sensor_DATA/17(V_eRR)
  Velocity_eRL [rad/s]/1 -> Sensor_DATA/18("V_eRL ")
  Constraints/1(Tq_FRout) -> Terminator/1
  Constraints/2("Tq_FLout ") -> Terminator1/1
  In_Numbers/4(Cornering Kamm_Factor [0-2]) -> [CK_Factor]
  [Re] -> Wheel_to_engine/5(Re)
  [RT] -> Wheel_to_engine/6(RT)
  Merge3/1 -> Display2/1, MaxFx_RL [N] (0,inf)/1, Wheel_to_engine/4("Fx_RL ")
  Merge2/1 -> MaxFx_RR [N] (0,inf)/1, Wheel_to_engine/3("Fx_RR "), Display4/1
  Merge1/1 -> Wheel_to_engine/2("Fx_FL ")
  Max Regen Torque [Nm]/1 -> In_Numbers/3(Max Regen Torque [Nm])
  Limit Power [kW]/1 -> In_Numbers/4(Limit Power [kW])
  Limit TemperatureIGBT/1 -> In_Numbers/5(Limit TemperatureIGBT [ºC])
  Reduction Power/1 -> In_Numbers/7(Reduction_P [0-1])
  [CK_Factor] -> Lateral Dynamics/13(CK_Factor)
  [SK_Factor] -> Longitudinal Dynamics/10(SK_Factor)
  Longitudinal Dynamics/1(Fx_FR) -> Merge/1
  Longitudinal Dynamics/2(Fx_FL) -> Merge1/1
  Longitudinal Dynamics/3("Fx_RR ") -> Merge2/1
  Longitudinal Dynamics/4("Fx_RL ") -> Merge3/1
  Merge/1 -> Wheel_to_engine/1("Fx_FR ")
  Steering Saturation (per site) [deg]/1 -> In_Numbers/9(Steering Saturation (per site) [deg])
  Ap_Sat_Up [-]/1 -> In_Numbers/10(Ap_Sat_Up [-])
  Ap_Sat_Down [-]/1 -> In_Numbers/11(Ap_Sat_Down [-])
  [MaxRegTorque] -> Constraints/18(MaxRegTorque)
  [ei_Perform] -> Terminator2/1
  Merge4/1 -> Mass [kg] (0,inf)/1
  Lateral Dynamics/6(" Mass [kg] (0,inf)") -> Merge4/2
  Lateral Dynamics/7(Handling [-] (-inf,inf)) -> Merge5/2
  Merge5/1 -> Handling [-] (-inf,inf)/1
  Merge6/1 -> Fy_R [N] (0,inf)/1
  Lateral Dynamics/5(Fy_R [N] (0,inf)) -> Merge6/2
  In_Numbers/16(ReductionCte_Temperature (0-1)) -> [ReductionCte_Temperature]
  Reduction Temperature/1 -> In_Numbers/8(Reduction_T [0-1])
  [ReductionCte_Temperature] -> Constraints/10(ReductionCte_Temperature)
  Constraints/3(Tq_RRout) -> Tq_RR [Nm] (0,inf)/1  "Out_RR"
  Constraints/4(Tq_RLout) -> Tq_RL [Nm] (0,inf)/1  "Out_RL"
  Temperature Motor [ºC]/1 -> Sensor_DATA/16(Temperature Motor)
  Sensor_DATA/15(TemperatureIGBT) -> [TemperatureIGBT]
  Sensor_DATA/16(TemperatureMotor) -> [TemperatureMotor]
  [TemperatureMotor] -> Constraints/13(TemperatureIMotor)
  [Temperature_limit_Motor] -> Constraints/12(TemperatureI_limit_Motor)
  In_Numbers/14(Temperature limit Motor [ºC]) -> [Temperature_limit_Motor]
  Limit TemperatureMotor/1 -> In_Numbers/6(Limit Temperature Motor [ºC])
  Merge7/1 -> [Flag_CarBehavior]
  Lateral Dynamics/8(Flag CarBehavior) -> Merge7/2
  MATLAB Function2/1(value) -> [Flag_WheelSpin_RL]
  MATLAB Function1/1(value) -> [Flag_WheelSpin_RR]
  Constant/1 -> MATLAB Function1/1(cte), MATLAB Function2/1(cte)
  Constraints/5(Flag_Temperature) -> [Flag_Temperature]
  Constraints/6(Flag_Power) -> [Flag_Power]
  Flags/1(Flags) -> Flags_[num5]/1
  [Flag_WheelSpin_RL] -> Flags/3(Flag_WheelSpin_RL)
  [Flag_WheelSpin_RR] -> Flags/2(Flag_WheelSpin_RR)
  [Flag_CarBehavior] -> Flags/1(Flag_CarBehavior)
  [Flag_Temperature] -> Flags/4(Flag_Temperature)
  [Flag_Power] -> Flags/5(Flag_Power)
  Optimization SKF & CKF/1(SKF_act) -> SKF_act/1, In_Numbers/1(S-Kamm_Factor)
  CKF_Initial/1 -> Optimization SKF & CKF/5(CKF_Initial)
  [Steer_An] -> Optimization SKF & CKF/3(Steer_An)
  [V_eRR] -> Optimization SKF & CKF/2(RPM_INV2)
  Cte_SKF/1 -> Optimization SKF & CKF/6(Cte_SKF)
  Cte_CKF/1 -> Optimization SKF & CKF/7(Cte_CKF)
  SKF_Initial/1 -> Optimization SKF & CKF/4(SKF_Initial)
  [V_eRL] -> Optimization SKF & CKF/1(RPM_INV1)
  Optimization SKF & CKF/2(CKF_act) -> CKF_act/1, In_Numbers/2(C-Kamm_Factor)
  Yaw_Rate [rad/s]/1 -> Sensor_DATA/5(Yaw Rate)
  Wheel_to_engine/1(Tq_diff) -> [Tq_diff]
  [Tq_diff] -> Constraints/21(Tq_diff)
  Sensor_DATA/5(YawRate) -> Lateral Dynamics/5(Yaw_Rate)
  Ellipse_acc/1 -> Sensor_DATA/4(Ellipse_acc)
  Gyro_Ellipse/1 -> Sensor_DATA/6(Gyro_Ellipse)
  Sensor_DATA/6(GyroEllipse) -> Lateral Dynamics/6(GyroEllipse)
  Sensor_DATA/4(Ellipse_Acc) -> Lateral Dynamics/4(Ellipse_Acc), Longitudinal Dynamics/3(Ellipse_Acc)
  In_Numbers/19(Yaw_error_correction_time [s]) -> [Yaw_error_correction_time]
  In_Numbers/18(Tq_diff_Max [Nm]) -> [Tq_diff_Max]
  [Yaw_error_correction_time] -> Lateral Dynamics/14(Yaw_error_/dt [s])
  [Ap] -> Longitudinal Dynamics/8(Gas_pedal)
  [Bp] -> Longitudinal Dynamics/9(Brake_pedal)
  Longitudinal Dynamics/6(Mass [kg] (0,inf)) -> [Mass_Recta]
  Longitudinal Dynamics/7(Handling [-] (-inf,inf)) -> [Handling_Recta]
  Longitudinal Dynamics/8(Flag CarBehavior) -> [Flag_BehaviourRecta]
  Longitudinal Dynamics/5(Fy_R) -> [Fy_R_Recta]
  [Fy_R_Recta] -> Merge6/1
  [Mass_Recta] -> Merge4/1
  [Handling_Recta] -> Merge5/1
  [Flag_BehaviourRecta] -> Merge7/1
  Lateral Dynamics/1(Fx_FR) -> [Fx_FR_Curva]
  Lateral Dynamics/2(Fx_FL) -> [Fx_FL_Curva]
  Lateral Dynamics/3("Fx_RR ") -> [Fx_RR_Curva]
  Lateral Dynamics/4("Fx_RL ") -> [Fx_RL_Curva]
  [Fx_FR_Curva] -> Merge/2
  [Fx_FL_Curva] -> Merge1/2
  [Fx_RR_Curva] -> Merge2/2
  [Fx_RL_Curva] -> Merge3/2
  Ellipse_vx/1 -> Sensor_DATA/19(Ellipse_vx)
  Sensor_DATA/19(Ellipse_Vx) -> Lateral Dynamics/15(Ellipse_Vx)
  [Tq_diff_Max] -> Constraints/22(Tq_diff_max)
  Temp_Celdas/1 -> Sensor_DATA/20(Temp_Celdas)
  Limit_Temp_Celdas/1 -> Sensor_DATA/21(Limit_Temp_Celdas)
  Sensor_DATA/20(Temp_celdas) -> [Temp_celdas]
  Sensor_DATA/21(Limit_Temp_celdas) -> [Limit_Temp_celdas]
  [Temp_celdas] -> Constraints/23(Temp_celdas)
  [Limit_Temp_celdas] -> Constraints/24(Limit_Temp_celdas)

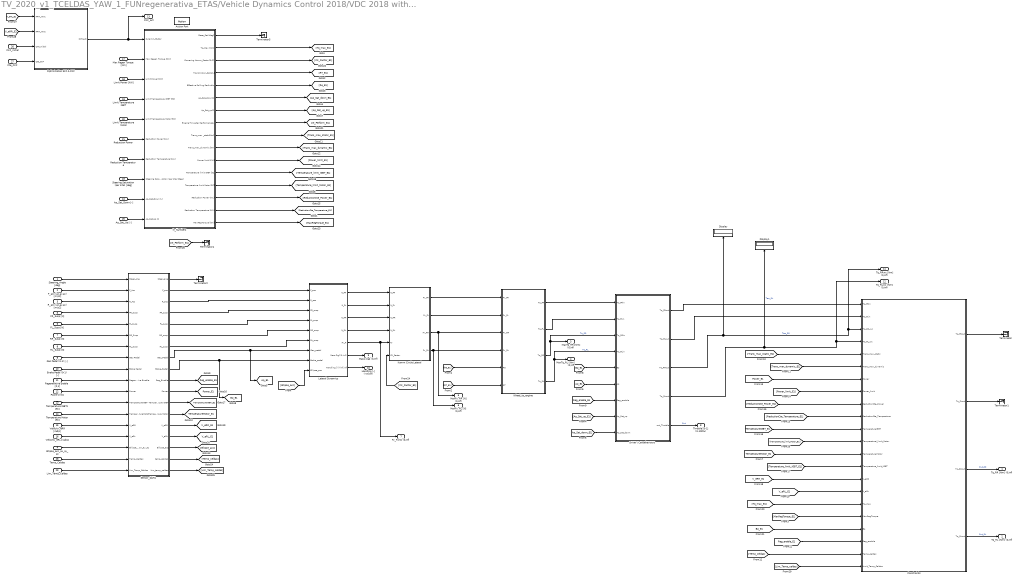
== system TV_2020_v1_TCELDAS_YAW_1_FUNregenerativa_ETAS/Vehicle Dynamics Control 2018/VDC 2018 without Longitudinal ==
  Steering_Angle [deg] : Inport
  F_acc (ax,ay,az) [m/s2] : Inport  Port=2
  R_acc (ax,ay,az) [m/s2] : Inport  Port=3
  Ellipse_acc_ax_ay_az : Inport  Port=4
  FR_Susp [N] : Inport  Port=5
  FL_Susp [N] : Inport  Port=6
  RR_Susp [N] : Inport  Port=7
  RL_Susp [N] : Inport  Port=8
  Gas Pedal (0-1) [-] : Inport  Port=9
  Brake Pedal (0-1) [-] : Inport  Port=10
  Regenerative Enable [0,1] : Inport  Port=11
  Power [kW] : Inport  Port=12
  Temperature IGBTs [ºC] : Inport  Port=13
  Temperature Motor [ºC] : Inport  Port=14
  Velocity_eRR [rad/s] : Inport  Port=15
  Velocity_eRL [rad/s] : Inport  Port=16
  Max Regen Torque [Nm] : Inport  Port=17
  Limit Power [kW] : Inport  Port=18
  Limit Temperature IGBT : Inport  Port=19
  Limit Temperature Motor : Inport  Port=20
  Reduction Power : Inport  Port=21
  Reduction Temperature : Inport  Port=22
  Steering Saturation (per site) [deg] : Inport  Port=23
  Ap_Sat_Down [-] : Inport  Port=24
  Ap_Sat_Up [-] : Inport  Port=25
  CKF_Initial : Inport  Port=26
  Cte_CKF : Inport  Port=27
  Temp_Celdas : Inport  Port=28
  Lim_Temp_Celdas : Inport  Port=29
  Action Port : ActionPort
  Constraints : Subsystem
  Display : Display
  Display1 : Display
  Driver / CarBehaviours : Subsystem
  In_Numbers : Subsystem
  Kamm Circle Lateral : Subsystem
  Lateral Dynamics : Subsystem
  Optimization SKF & CKF : Subsystem
  Sensor_DATA : Subsystem
  Terminator{,1..2,4..5} (5 alike) : Terminator
  Wheel_to_engine : Subsystem
  Tq_RR [Nm] (0,inf) : Outport
  Tq_RL [Nm] (0,inf) : Outport  Port=2
  MaxTq_RR [Nm] (0,inf) : Outport  Port=3
  MaxTq_RL [Nm] (0,inf) : Outport  Port=4
  MaxFx_RR [N] (0,inf) : Outport  Port=5
  MaxFx_RL [N] (0,inf) : Outport  Port=6
  Fy_R [N] (0,inf) : Outport  Port=7
  Throttle [0-1] (0-100%) : Outport  Port=8
  Mass [kg] (0,inf) : Outport  Port=9
  Handling [-] (-inf,inf) : Outport  Port=10
  Tq_RRwc [Nm] (0,inf) : Outport  Port=11
  Tq_RLwc [Nm] (0,inf) : Outport  Port=12
  CKF_act : Outport  Port=13
  tag scope: Ap_E1=global, Bp_E1=global, Power_E1=global, Reg_enable_E1=global, TemperatureIGBT_E1=global, TemperatureMotor_E1=global, V_eRL_E1=global, V_eRR_E1=global
  wires:
  Sensor_DATA/7(RL_susp) -> Lateral Dynamics/6(RL_susp)
  In_Numbers/2(Tq_Max [Nm]) -> [Tq_max_E1]
  Sensor_DATA/8(Gas_Pedal) -> [Ap_E1], Lateral Dynamics/7(Gas_pedal)
  In_Numbers/5(Effective Rolling Radius[m]) -> [Re_E1]
  In_Numbers/4(Transmision_Ratio[-]) -> [RT_E1]
  Sensor_DATA/6(RR_susp) -> Lateral Dynamics/5(RR_susp)
  In_Numbers/7(Ap_Sat_up[-]) -> [Ap_Sat_up_E1]
  In_Numbers/6(Ap_Sat_down[-]) -> [Ap_Sat_down_E1]
  Sensor_DATA/2(F_acc) -> Lateral Dynamics/1(F_acc)
  Sensor_DATA/3(R_acc) -> Lateral Dynamics/2(R_acc)
  Sensor_DATA/9(Brake_Pedal) -> [Bp_E1], Lateral Dynamics/8(Brake_pedal)
  Sensor_DATA/5(FL_susp) -> Lateral Dynamics/4(FL_susp)
  Sensor_DATA/10(Reg_Enable) -> [Reg_enable_E1]
  Sensor_DATA/4(FR_susp) -> Lateral Dynamics/3(FR_susp)
  Wheel_to_engine/4(Tq_RL) -> Driver / CarBehaviours/4("Tq_RLin "), MaxTq_RL [Nm] (0,inf)/1  "Tq_RL"
  In_Numbers/14(Reduction Power (0-1)) -> [ReductionCte_Power_E1]
  Wheel_to_engine/3(Tq_RR) -> MaxTq_RR [Nm] (0,inf)/1, Driver / CarBehaviours/3(Tq_RRin)  "Tq_RR"
  Wheel_to_engine/2(Tq_FL) -> Driver / CarBehaviours/2(Tq_FLin)
  In_Numbers/10(Trans_max_dynamic [Nm]) -> [Trans_max_dynamic_E1]
  [Reg_enable_E1] -> Driver / CarBehaviours/7(Reg_enable)
  [Ap_Sat_up_E1] -> Driver / CarBehaviours/8(Ap_Sat_up)
  In_Numbers/9(Trans_max _static[Nm]) -> [Trans_max_static_E1]
  [Ap_E1] -> Driver / CarBehaviours/6(Ap)
  In_Numbers/11("Power limit [KW] ") -> [Power_limit_E1]
  [Ap_Sat_down_E1] -> Driver / CarBehaviours/9(Ap_Sat_down)
  Steering_Angle [deg]/1 -> Sensor_DATA/1(Steer_Ang)
  Wheel_to_engine/1(Tq_FR) -> Driver / CarBehaviours/1(Tq_FRin)
  Sensor_DATA/15(V_eRL) -> [V_eRL_E1]
  In_Numbers/16(MaxRegTorque [Nm]) -> [MaxRegTorque_E1]
  In_Numbers/8(Engine+Inverter Performance[-]) -> [ei_Perform_E1]
  [Bp_E1] -> Driver / CarBehaviours/5(Bp)
  Sensor_DATA/12(Temperature IGBT) -> [TemperatureIGBT_E1]
  RR_Susp [N]/1 -> Sensor_DATA/6(RR_Susp)
  Power [kW]/1 -> Sensor_DATA/11("Power ")
  Sensor_DATA/11(Power) -> [Power_E1]
  Sensor_DATA/14("V_eRR ") -> [V_eRR_E1]
  Regenerative Enable [0,1]/1 -> Sensor_DATA/10(Regenerative Enable)
  Brake Pedal (0-1) [-]/1 -> Sensor_DATA/9(Brake Pedal)
  In_Numbers/12(Temperature limit IGBT [ºC]) -> [Temperature_limit_IGBT_E1]
  FL_Susp [N]/1 -> Sensor_DATA/5(FL_Susp)
  FR_Susp [N]/1 -> Sensor_DATA/4(FR_Susp)
  R_acc (ax,ay,az) [m/s2]/1 -> Sensor_DATA/3(R_Acc)
  F_acc (ax,ay,az) [m/s2]/1 -> Sensor_DATA/2("F_Acc ")
  RL_Susp [N]/1 -> Sensor_DATA/7(RL_Susp)
  Gas Pedal (0-1) [-]/1 -> Sensor_DATA/8(Gas Pedal)
  Temperature IGBTs [ºC]/1 -> Sensor_DATA/12(TemperatureIGBT)
  Velocity_eRR [rad/s]/1 -> Sensor_DATA/14(V_eRR)
  Velocity_eRL [rad/s]/1 -> Sensor_DATA/15("V_eRL ")
  Max Regen Torque [Nm]/1 -> In_Numbers/2(Max Regen Torque [Nm])
  Limit Power [kW]/1 -> In_Numbers/3(Limit Power [kW])
  Limit Temperature IGBT/1 -> In_Numbers/4(Limit Temperature IGBT [ºC])
  Reduction Power/1 -> In_Numbers/6(Reduction Power [0-1])
  In_Numbers/3(Cornering Kamm_Factor [0-2]) -> [CK_Factor_E1]
  [Re_E1] -> Wheel_to_engine/5(Re)
  [RT_E1] -> Wheel_to_engine/6(RT)
  Ap_Sat_Up [-]/1 -> In_Numbers/10(Ap_Sat_Up [-])
  Ap_Sat_Down [-]/1 -> In_Numbers/9(Ap_Sat_Down [-])
  Steering Saturation (per site) [deg]/1 -> In_Numbers/8(Steering Saturation (per site) [deg])
  [CK_Factor_E1] -> Kamm Circle Lateral/6(CK_Factor)
  Kamm Circle Lateral/1(Fx_FR) -> Wheel_to_engine/1("Fx_FR ")
  Kamm Circle Lateral/2(Fx_FL) -> Wheel_to_engine/2("Fx_FL ")
  Kamm Circle Lateral/3("Fx_RR ") -> MaxFx_RR [N] (0,inf)/1, Wheel_to_engine/3("Fx_RR ")
  Kamm Circle Lateral/4("Fx_RL ") -> MaxFx_RL [N] (0,inf)/1, Wheel_to_engine/4("Fx_RL ")
  Sensor_DATA/1(Steer_ang) -> Terminator2/1
  Lateral Dynamics/1(N_FR) -> Kamm Circle Lateral/1("N_FR ")
  Lateral Dynamics/2("N_FL ") -> Kamm Circle Lateral/2(N_FL)
  Lateral Dynamics/3("N_RR ") -> Kamm Circle Lateral/3(N_RR)
  Lateral Dynamics/4(N_RL) -> Kamm Circle Lateral/4(N_RL)
  Driver / CarBehaviours/5(out_Throttle) -> Throttle [0-1] (0-100%)/1  "Out"
  [ei_Perform_E1] -> Terminator4/1
  In_Numbers/1(Steer_Sat [deg]) -> Terminator5/1
  Lateral Dynamics/6(Mass [kg] (0,inf)) -> Mass [kg] (0,inf)/1
  Lateral Dynamics/7(Handling [-] (-inf,inf)) -> Handling [-] (-inf,inf)/1
  In_Numbers/15(Reduction Temperature (0-1)) -> [ReductionCte_Temperature_E1]
  Reduction Temperature/1 -> In_Numbers/7(Reduction Temperature [0-1])
  Driver / CarBehaviours/3(Tq_RRout) -> Tq_RRwc [Nm] (0,inf)/1, Constraints/3(Tq_RR_wc), Display/1  "Teo_RR"
  [Trans_max_dynamic_E1] -> Constraints/6(Trans_max_dynamic)
  [Power_limit_E1] -> Constraints/8(Power_limit)
  [ReductionCte_Power_E1] -> Constraints/9(ReductionCte_Power)
  [Power_E1] -> Constraints/7(Power)
  Driver / CarBehaviours/4(Tq_RLout) -> Tq_RLwc [Nm] (0,inf)/1, Constraints/4("Tq_RL_wc "), Display1/1  "Teo_RL"
  Driver / CarBehaviours/2("Tq_FLout ") -> Constraints/2(Tq_FLin)
  Driver / CarBehaviours/1(Tq_FRout) -> Constraints/1(Tq_FRin)
  [Trans_max_static_E1] -> Constraints/5("Trans_max_static ")
  [Temperature_limit_IGBT_E1] -> Constraints/14(Temperature_limit_IGBT)
  [Bp_E1] -> Constraints/19(Bp)
  [TemperatureIGBT_E1] -> Constraints/11(TemperatureIGBT)
  [Reg_enable_E1] -> Constraints/20(Reg_enable)
  [Tq_max_E1] -> Constraints/17(Tq_max)
  [V_eRR_E1] -> Constraints/15(V_eRR)
  [V_eRL_E1] -> Constraints/16(V_eRL)
  Constraints/1(Tq_FRout) -> Terminator/1
  Constraints/2("Tq_FLout ") -> Terminator1/1
  [MaxRegTorque_E1] -> Constraints/18(MaxRegTorque)
  [ReductionCte_Temperature_E1] -> Constraints/10(ReductionCte_Temperature)
  [TemperatureMotor_E1] -> Constraints/13(TemperatureIMotor)
  [Temperature_limit_Motor_E1] -> Constraints/12(TemperatureI_limit_Motor)
  Limit Temperature Motor/1 -> In_Numbers/5(Limit Temperature Motor [ºC])
  In_Numbers/13(Temperature limit Motor [ºC]) -> [Temperature_limit_Motor_E1]
  Temperature Motor [ºC]/1 -> Sensor_DATA/13(TemperatureMotor)
  Sensor_DATA/13(Temperature Motor) -> [TemperatureMotor_E1]
  [V_eRR_E1] -> Optimization SKF & CKF/2(RPM_INV2)
  CKF_Initial/1 -> Optimization SKF & CKF/3(CKF_Initial)
  Cte_CKF/1 -> Optimization SKF & CKF/4(Cte_CKF)
  Optimization SKF & CKF/1(CKF_act) -> CKF_act/1, In_Numbers/1(C-Kamm_Factor)
  [V_eRL_E1] -> Optimization SKF & CKF/1(RPM_INV1)
  Constraints/3(Tq_RRout) -> Tq_RR [Nm] (0,inf)/1  "Out_RR"
  Constraints/4(Tq_RLout) -> Tq_RL [Nm] (0,inf)/1  "Out_RL"
  Ellipse_acc_ax_ay_az/1 -> Sensor_DATA/16(Ellipse_acc_ax_ay_az)
  Sensor_DATA/16(Ellipse_acc) -> [Ellipse_acc]
  Lateral Dynamics/5(Fy_R) -> Kamm Circle Lateral/5(Fy), Fy_R [N] (0,inf)/1
  [Ellipse_acc] -> Lateral Dynamics/9(Ellipse_acc)
  Temp_Celdas/1 -> Sensor_DATA/17(Temp_Celdas)
  Lim_Temp_Celdas/1 -> Sensor_DATA/18(Lim_Temp_Celdas)
  Sensor_DATA/17(temp_celdas) -> [Temp_celdas]
  Sensor_DATA/18(Lim_temp_celdas) -> [Lim_Temp_celdas]
  [Temp_celdas] -> Constraints/21(Temp_celdas)
  [Lim_Temp_celdas] -> Constraints/22(Limit_Temp_Celdas)

== system TV_2020_v1_TCELDAS_YAW_1_FUNregenerativa_ETAS/Vehicle Dynamics Control 2018/Rigid Axle/Accelerating ==
  Ap : Inport
  "Ap_Sat_up " : Inport  Port=2
  Ap_Sat_down : Inport  Port=3
  Tq_RR : Inport  Port=4
  "Tq_RL " : Inport  Port=5
  "Accelerator behaviour " : MATLAB Function  TreatAsAtomicUnit=on
  Product : Product
  Product1 : Product
  "Tq_RR " : Outport
  Tq_RL : Outport  Port=2
  wires:
  Ap_Sat_down/1 -> "Accelerator behaviour "/3(Ap_Sat_down)
  Product/1 -> Tq_RL/1
  "Accelerator behaviour "/1(throttle) -> Product/1, Product1/1
  "Ap_Sat_up "/1 -> "Accelerator behaviour "/2(Ap_Sat_up)
  Ap/1 -> "Accelerator behaviour "/1(Ap)
  Tq_RR/1 -> Product1/2
  "Tq_RL "/1 -> Product/2
  Product1/1 -> "Tq_RR "/1

== system TV_2020_v1_TCELDAS_YAW_1_FUNregenerativa_ETAS/Vehicle Dynamics Control 2018/Steering TV 2017 with TC/Accelerating ==
  Ap : Inport
  "Ap_Sat_up " : Inport  Port=2
  Ap_Sat_down : Inport  Port=3
  Tq_RR : Inport  Port=4
  "Tq_RL " : Inport  Port=5
  "Accelerator behaviour " : MATLAB Function  TreatAsAtomicUnit=on
  Product : Product
  Product1 : Product
  "Tq_RR " : Outport
  Tq_RL : Outport  Port=2
  wires:
  Ap_Sat_down/1 -> "Accelerator behaviour "/3(Ap_Sat_down)
  Product/1 -> Tq_RL/1
  "Accelerator behaviour "/1(throttle) -> Product/1, Product1/1
  "Ap_Sat_up "/1 -> "Accelerator behaviour "/2(Ap_Sat_up)
  Ap/1 -> "Accelerator behaviour "/1(Ap)
  Tq_RR/1 -> Product1/2
  "Tq_RL "/1 -> Product/2
  Product1/1 -> "Tq_RR "/1

== system TV_2020_v1_TCELDAS_YAW_1_FUNregenerativa_ETAS/Vehicle Dynamics Control 2018/Steering TV 2017 with TC/Constraints ==
  note: Considero de la misma gravedad,
      | la limitacion por potencia que por temperatura
  Power_limit : Inport
  Power : Inport  Port=2
  Temperature_limit_IGBT : Inport  Port=3
  Temperature_IGBT : Inport  Port=4
  Temperature_limit_Motor : Inport  Port=5
  Temperature_Motor : Inport  Port=6
  Temp_Celdas : Inport  Port=7
  Lim_Temp_Celdas : Inport  Port=8
  Tq_RR : Inport  Port=9
  Tq_RL : Inport  Port=10
  ReductionCte_Temperature : Inport  Port=11
  ReductionCte_Power : Inport  Port=12
  "Control de Potencia " : Subsystem  TreatAsAtomicUnit=on
  Control de Temperatura : Subsystem  TreatAsAtomicUnit=on
  If : If  NumInputs=8  IfExpression=u4 >= u3 | u6 >= u5 | u7>=u8  ElseIfExpressions=u2 >= u1
  Merge : Merge  Inputs=3
  Merge1 : Merge  Inputs=3
  else : Subsystem  TreatAsAtomicUnit=on
  TQ_RR : Outport
  TQ_RL : Outport  Port=2
  wires:
  ReductionCte_Power/1 -> "Control de Potencia "/3(ReductionCte)
  Power_limit/1 -> If/1
  Temperature_limit_IGBT/1 -> If/3
  ReductionCte_Temperature/1 -> Control de Temperatura/3(ReductionCte)
  Power/1 -> If/2
  "Control de Potencia "/1(Tq_RR_out) -> Merge/1
  "Control de Potencia "/2(Tq_RL_out) -> Merge1/1
  else/2(Tq_RL_out) -> Merge1/3
  If/1 -> Control de Temperatura/Action
  Tq_RR/1 -> else/1(Tq_RR), Control de Temperatura/1(Tq_RR), "Control de Potencia "/1(Tq_RR)
  Tq_RL/1 -> Control de Temperatura/2(Tq_RL), "Control de Potencia "/2(Tq_RL), else/2(Tq_RL)
  If/2 -> "Control de Potencia "/Action
  If/3 -> else/Action
  Control de Temperatura/1(Tq_RR_out) -> Merge/2
  else/1(Tq_RR_out) -> Merge/3
  Control de Temperatura/2(Tq_RL_out) -> Merge1/2
  Temperature_limit_Motor/1 -> If/5
  Temperature_Motor/1 -> If/6
  Merge/1 -> TQ_RR/1
  Merge1/1 -> TQ_RL/1
  Temperature_IGBT/1 -> If/4
  Temp_Celdas/1 -> If/7
  Lim_Temp_Celdas/1 -> If/8

== system TV_2020_v1_TCELDAS_YAW_1_FUNregenerativa_ETAS/Vehicle Dynamics Control 2018/Steering TV 2017 with TC/Lateral Dynamics ==
  CKF : Inport
  Tq_RR : Inport  Port=2
  Tq_RL : Inport  Port=3
  Action Port : ActionPort
  Product : Product
  Product1 : Product
  Tq_RR_with_CKF : Outport
  Tq_RL_with_CKF : Outport  Port=2
  wires:
  Product1/1 -> Tq_RL_with_CKF/1
  Tq_RR/1 -> Product/1
  Tq_RL/1 -> Product1/1
  CKF/1 -> Product/2, Product1/2
  Product/1 -> Tq_RR_with_CKF/1

== system TV_2020_v1_TCELDAS_YAW_1_FUNregenerativa_ETAS/Vehicle Dynamics Control 2018/Steering TV 2017 with TC/Longitudinal Dynamics ==
  SKF : Inport
  Tq_RR : Inport  Port=2
  Tq_RL : Inport  Port=3
  Action Port : ActionPort
  Product : Product
  Product1 : Product
  Tq_RR_with_SKF : Outport
  Tq_RL_with_SKF : Outport  Port=2
  wires:
  Tq_RR/1 -> Product/1
  Tq_RL/1 -> Product1/1
  SKF/1 -> Product/2, Product1/2
  Product/1 -> Tq_RR_with_SKF/1
  Product1/1 -> Tq_RL_with_SKF/1
